simulink model "SimulinkArduino"  (R2023b)
settings: Solver=VariableStepAuto  StartTime=0.0  StopTime=10.0  RelTol=1e-3
values from neighbouring files (symbols this model uses):
  Hf = tf(2,conv([1,1],[10,1]),'iodelay',1)    [IRA2Laborator2.m]
libraries: instrumentseriallib x3
settings Model: Creator=receaalex  LastModifiedBy=receaalex

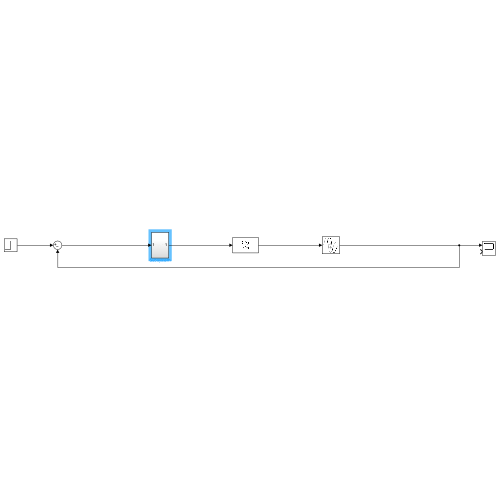
[thumbnail: Simulink's stored preview of the top-level diagram]
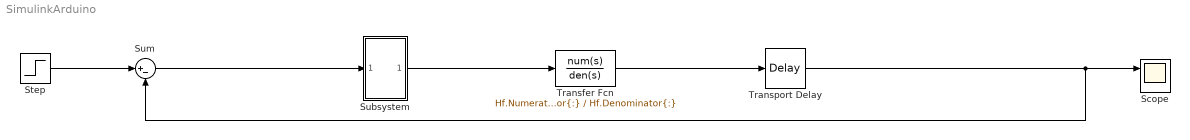
== system SimulinkArduino ==
  Scope : Scope  NumInputPorts=2
  Step : Step  SampleTime=0
  Subsystem : Subsystem
  Sum : Sum  Inputs=|+-
  Transfer Fcn : TransferFcn  Numerator=Hf.Numerator{:}  Denominator=Hf.Denominator{:}
  Transport Delay : TransportDelay
  wires:
  Transfer Fcn/1 -> Transport Delay/1
  Step/1 -> Sum/1
  Transport Delay/1 -> Sum/2, Scope/1
  Sum/1 -> Subsystem/1(In1)
  Subsystem/1(Out1) -> Transfer Fcn/1

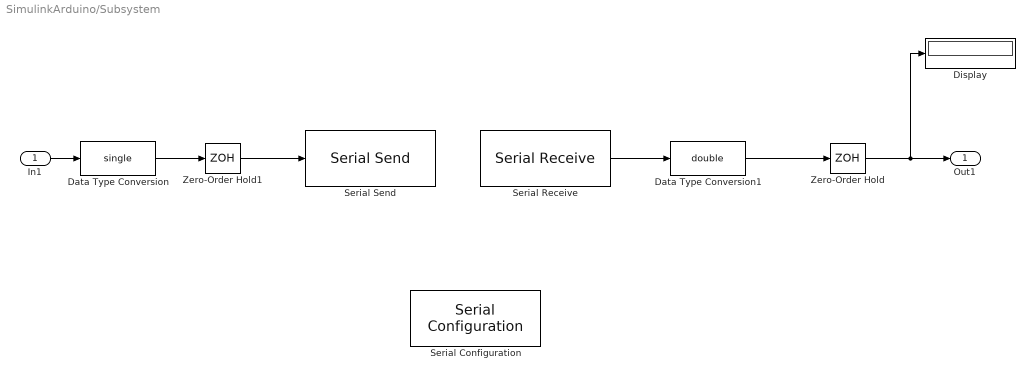
== system SimulinkArduino/Subsystem ==
  In1 : Inport
  Data Type Conversion : DataTypeConversion  OutDataTypeStr=single  SaturateOnIntegerOverflow=off  RndMeth=Floor
  Data Type Conversion1 : DataTypeConversion  OutDataTypeStr=double  SaturateOnIntegerOverflow=off  RndMeth=Floor
  Display : Display
  Serial Configuration : instrumentseriallib/Serial Configuration  Priority=-200000  PortSel=<Select a port...>  Port=<Select a port...>  ComPort=<Select a port...>  BaudRate=9600  DataBits=8  Parity=none  StopBits=1  ByteOrder=little-endian  FlowControl=none  Timeout=10  SimulateUsing=Interpreted execution  BlockInModel=on  aMode=1
  Serial Receive : instrumentseriallib/Serial Receive  Priority=1  PortSel=<Select a port...>  Port=<Select a port...>  ComPort=<Select a port...>  DataType=single  SaveDataType=uint8  ToggleHeader=off  Header=[]  ToggleTerminator=off  Terminator=<none>  CustomTerminator=[]  InputFormat=Column major  ToggleDataSize=on  DataSize=[1 1]  EnableBlockingMode=on  ActionDataUnavailable=Output last received value  ActionWhenDataUnavailable=Output last received value  CustomValue=0  SampleTime=0.2  SimulateUsing=Interpreted execution  BlockInModel=on  aMode=1
  Serial Send : instrumentseriallib/Serial Send  Priority=1  PortSel=<Select a port...>  Port=<Select a port...>  ComPort=<Select a port...>  Header=[]  Terminator=<none>  CustomTerminator=[]  EnableBlockingMode=on  SimulateUsing=Interpreted execution  BlockInModel=on  aMode=1
  Zero-Order Hold : ZeroOrderHold  SampleTime=-1
  Zero-Order Hold1 : ZeroOrderHold  SampleTime=-1
  Out1 : Outport
  wires:
  Serial Receive/1 -> Data Type Conversion1/1
  In1/1 -> Data Type Conversion/1
  Data Type Conversion/1 -> Zero-Order Hold1/1
  Data Type Conversion1/1 -> Zero-Order Hold/1
  Zero-Order Hold/1 -> Display/1, Out1/1
  Zero-Order Hold1/1 -> Serial Send/1
